simulink model "lqe_h"  (R2020b)
settings: Solver=VariableStepAuto  StartTime=0.0  StopTime=10.0  RelTol=1e-3
settings Model: Creator=leonk  LastModifiedBy=leonk

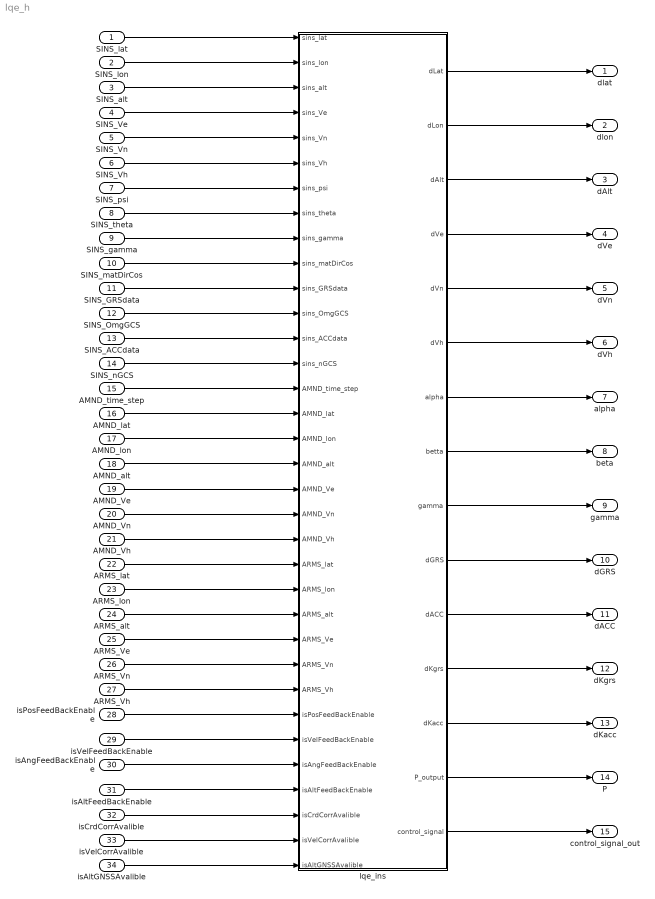
== system lqe_h ==
  SINS_lat : Inport  PortDimensions=1
  SINS_lon : Inport  Port=2  PortDimensions=1
  SINS_alt : Inport  Port=3  PortDimensions=1
  SINS_Ve : Inport  Port=4  PortDimensions=1
  SINS_Vn : Inport  Port=5  PortDimensions=1
  SINS_Vh : Inport  Port=6  PortDimensions=1
  SINS_psi : Inport  Port=7  PortDimensions=1
  SINS_theta : Inport  Port=8  PortDimensions=1
  SINS_gamma : Inport  Port=9  PortDimensions=1
  SINS_matDirCos : Inport  Port=10  PortDimensions=[3,3]
  SINS_GRSdata : Inport  Port=11  PortDimensions=[3,1]
  SINS_OmgGCS : Inport  Port=12  PortDimensions=[3,1]
  SINS_ACCdata : Inport  Port=13  PortDimensions=[3,1]
  SINS_nGCS : Inport  Port=14  PortDimensions=[3,1]
  AMND_time_step : Inport  Port=15  PortDimensions=1
  AMND_lat : Inport  Port=16  PortDimensions=1
  AMND_lon : Inport  Port=17  PortDimensions=1
  AMND_alt : Inport  Port=18  PortDimensions=1
  AMND_Ve : Inport  Port=19  PortDimensions=1
  AMND_Vn : Inport  Port=20  PortDimensions=1
  AMND_Vh : Inport  Port=21  PortDimensions=1
  ARMS_lat : Inport  Port=22  PortDimensions=1
  ARMS_lon : Inport  Port=23  PortDimensions=1
  ARMS_alt : Inport  Port=24  PortDimensions=1
  ARMS_Ve : Inport  Port=25  PortDimensions=1
  ARMS_Vn : Inport  Port=26  PortDimensions=1
  ARMS_Vh : Inport  Port=27  PortDimensions=1
  isPosFeedBackEnable : Inport  Port=28  PortDimensions=1
  isVelFeedBackEnable : Inport  Port=29  PortDimensions=1
  isAngFeedBackEnable : Inport  Port=30  PortDimensions=1
  isAltFeedBackEnable : Inport  Port=31  PortDimensions=1
  isCrdCorrAvalible : Inport  Port=32  PortDimensions=1
  isVelCorrAvalible : Inport  Port=33  PortDimensions=1
  isAltGNSSAvalible : Inport  Port=34  PortDimensions=1
  lqe_ins : MATLAB Function  TreatAsAtomicUnit=on
  dlat : Outport  PortDimensions=1  VectorParamsAs1DForOutWhenUnconnected=off
  dlon : Outport  Port=2  PortDimensions=1  VectorParamsAs1DForOutWhenUnconnected=off
  dAlt : Outport  Port=3  PortDimensions=1  VectorParamsAs1DForOutWhenUnconnected=off
  dVe : Outport  Port=4  PortDimensions=1  VectorParamsAs1DForOutWhenUnconnected=off
  dVn : Outport  Port=5  PortDimensions=1  VectorParamsAs1DForOutWhenUnconnected=off
  dVh : Outport  Port=6  PortDimensions=1  VectorParamsAs1DForOutWhenUnconnected=off
  alpha : Outport  Port=7  PortDimensions=1  VectorParamsAs1DForOutWhenUnconnected=off
  beta : Outport  Port=8  PortDimensions=1  VectorParamsAs1DForOutWhenUnconnected=off
  gamma : Outport  Port=9  PortDimensions=1  VectorParamsAs1DForOutWhenUnconnected=off
  dGRS : Outport  Port=10  PortDimensions=[3,1]  VectorParamsAs1DForOutWhenUnconnected=off
  dACC : Outport  Port=11  PortDimensions=[3,1]  VectorParamsAs1DForOutWhenUnconnected=off
  dKgrs : Outport  Port=12  PortDimensions=[3,1]  VectorParamsAs1DForOutWhenUnconnected=off
  dKacc : Outport  Port=13  PortDimensions=[3,1]  VectorParamsAs1DForOutWhenUnconnected=off
  P : Outport  Port=14  VectorParamsAs1DForOutWhenUnconnected=off
  control_signal_out : Outport  Port=15  PortDimensions=[4,1]  VectorParamsAs1DForOutWhenUnconnected=off
  wires:
  isAltFeedBackEnable/1 -> lqe_ins/31(isAltFeedBackEnable)
  lqe_ins/6(dVh) -> dVh/1
  AMND_lon/1 -> lqe_ins/17(AMND_lon)
  lqe_ins/9(gamma) -> gamma/1
  ARMS_Vn/1 -> lqe_ins/26(ARMS_Vn)
  lqe_ins/4(dVe) -> dVe/1
  SINS_alt/1 -> lqe_ins/3(sins_alt)
  isVelCorrAvalible/1 -> lqe_ins/33(isVelCorrAvalible)
  isCrdCorrAvalible/1 -> lqe_ins/32(isCrdCorrAvalible)
  lqe_ins/2(dLon) -> dlon/1
  AMND_Vn/1 -> lqe_ins/20(AMND_Vn)
  lqe_ins/5(dVn) -> dVn/1
  ARMS_Vh/1 -> lqe_ins/27(ARMS_Vh)
  lqe_ins/1(dLat) -> dlat/1
  AMND_alt/1 -> lqe_ins/18(AMND_alt)
  AMND_Vh/1 -> lqe_ins/21(AMND_Vh)
  lqe_ins/3(dAlt) -> dAlt/1
  ARMS_alt/1 -> lqe_ins/24(ARMS_alt)
  lqe_ins/8(betta) -> beta/1
  lqe_ins/13(dKacc) -> dKacc/1
  SINS_ACCdata/1 -> lqe_ins/13(sins_ACCdata)
  isPosFeedBackEnable/1 -> lqe_ins/28(isPosFeedBackEnable)
  lqe_ins/15(control_signal) -> control_signal_out/1
  AMND_time_step/1 -> lqe_ins/15(AMND_time_step)
  SINS_Ve/1 -> lqe_ins/4(sins_Ve)
  isVelFeedBackEnable/1 -> lqe_ins/29(isVelFeedBackEnable)
  AMND_Ve/1 -> lqe_ins/19(AMND_Ve)
  SINS_nGCS/1 -> lqe_ins/14(sins_nGCS)
  SINS_GRSdata/1 -> lqe_ins/11(sins_GRSdata)
  lqe_ins/10(dGRS) -> dGRS/1
  isAltGNSSAvalible/1 -> lqe_ins/34(isAltGNSSAvalible)
  SINS_Vh/1 -> lqe_ins/6(sins_Vh)
  ARMS_lon/1 -> lqe_ins/23(ARMS_lon)
  AMND_lat/1 -> lqe_ins/16(AMND_lat)
  isAngFeedBackEnable/1 -> lqe_ins/30(isAngFeedBackEnable)
  ARMS_Ve/1 -> lqe_ins/25(ARMS_Ve)
  ARMS_lat/1 -> lqe_ins/22(ARMS_lat)
  SINS_gamma/1 -> lqe_ins/9(sins_gamma)
  SINS_lat/1 -> lqe_ins/1(sins_lat)
  SINS_OmgGCS/1 -> lqe_ins/12(sins_OmgGCS)
  SINS_theta/1 -> lqe_ins/8(sins_theta)
  lqe_ins/12(dKgrs) -> dKgrs/1
  SINS_Vn/1 -> lqe_ins/5(sins_Vn)
  lqe_ins/11(dACC) -> dACC/1
  lqe_ins/14(P_output) -> P/1
  lqe_ins/7(alpha) -> alpha/1
  SINS_matDirCos/1 -> lqe_ins/10(sins_matDirCos)
  SINS_psi/1 -> lqe_ins/7(sins_psi)
  SINS_lon/1 -> lqe_ins/2(sins_lon)

== matlab function lqe_h/lqe_ins ==
  data: sins_lat input; sins_lon input; sins_alt input; sins_Ve input; sins_Vn input; sins_Vh input; sins_psi input; sins_theta input; sins_gamma input; sins_matDirCos input; sins_GRSdata input; sins_OmgGCS input; sins_ACCdata input; sins_nGCS input; AMND_time_step input; AMND_lat input; AMND_lon input; AMND_alt input; AMND_Ve input; AMND_Vn input; AMND_Vh input; ARMS_lat input; ARMS_lon input; ARMS_alt input; ARMS_Ve input; ARMS_Vn input; ARMS_Vh input; isPosFeedBackEnable input; isVelFeedBackEnable input; dLat output; dLon output; dAlt output; dVe output; dVn output; dVh output; alpha output; betta output; gamma output; dGRS output; dACC output; dKgrs output; dKacc output; isAngFeedBackEnable input; isAltFeedBackEnable input; P_output output; control_signal output; isCrdCorrAvalible input; isVelCorrAvalible input; isAltGNSSAvalible input
function [dLat,dLon,dAlt,dVe,dVn,dVh,alpha,betta,gamma,dGRS, dACC, dKgrs,dKacc,...
    P_output, control_signal]=...
    lqe_ins(...
    sins_lat, sins_lon, sins_alt, sins_Ve, sins_Vn, sins_Vh,sins_psi, sins_theta,...
    sins_gamma,sins_matDirCos, sins_GRSdata, sins_OmgGCS, sins_ACCdata,...
    sins_nGCS,...
    AMND_time_step,...
    AMND_lat, AMND_lon, AMND_alt, AMND_Ve, AMND_Vn, AMND_Vh,... 
    ARMS_lat, ARMS_lon,ARMS_alt, ARMS_Ve, ARMS_Vn, ARMS_Vh,...
    isPosFeedBackEnable, isVelFeedBackEnable, isAngFeedBackEnable, isAltFeedBackEnable,...
    isCrdCorrAvalible, isVelCorrAvalible, isAltGNSSAvalible)
   
    persistent LQE SINS AMND time 
    
    u = deg2rad(15/3600); 
    EARTH_A = 6378147;
    RO_1 = EARTH_A;
    RO_2 = EARTH_A;
    GRAVIT_CONST_EATRH = 3.9860e+14;
    EARTH_A = 6378147;
    SQR_OM_SH = (GRAVIT_CONST_EATRH/(EARTH_A*EARTH_A*EARTH_A));
    
    
    if isempty(LQE) 
        time = 0;
        LQE.Z = zeros(7,1);
        LQE.X = zeros(21,1);
        LQE.F = zeros(21,21);
        LQE.S = zeros(21,21);
        LQE.P = zeros(21,21);
        LQE.G = zeros(21,6);
        LQE.L = zeros(21,6);
        LQE.Q = zeros(6,6);
        LQE.K = zeros(21,7);
        LQE.R = zeros(7,7);
        LQE.H = zeros(7,21);
        LQE.prediction_step = 1/100;
        LQE.isPosFeedBackEnable = isPosFeedBackEnable;%0;%
        LQE.isVelFeedBackEnable = isVelFeedBackEnable;%0;%
        LQE.isAngFeedBackEnable = isAngFeedBackEnable;%0;%
        LQE.isAltFeedBackEnable = isAltFeedBackEnable;
        
        LQE.isCrdCorrAvalible   = 0;
        LQE.isVelCorrAvalible   = 0;
        LQE.isAltGNSSAvalible = 0;
        LQE.isCorrAvalible    = 0;
        
        LQE = init_PQ(LQE);
        
        SINS.lat   = 0;
        SINS.lon   = 0;
        SINS.alt   = 0;
        SINS.Ve    = 0;
        SINS.Vn    = 0;
        SINS.Vh    = 0;
        SINS.psi   = 0;
        SINS.theta = 0;
        SINS.gamma = 0;
        SINS.matDirCos = zeros(3,3);
        SINS.Omg_x = 0;
        SINS.Omg_y = 0;
        SINS.Omg_z = 0;
        SINS.Omg_e = 0;
        SINS.Omg_n = 0;
        SINS.Omg_h = 0;
        SINS.n_x   = 0;
        SINS.n_y   = 0;
        SINS.n_z   = 0;
        SINS.n_e   = 0;
        SINS.n_n   = 0;
        SINS.n_h   = 0;
        
        AMND.lat = 0;
        AMND.lon = 0;
        AMND.alt = 0;
        AMND.Ve  = 0;
        AMND.Vn  = 0;
        AMND.Vh = 0;
        AMND.lat_RMS = 0;
        AMND.lon_RMS = 0;
        AMND.alt_RMS = 0;
        AMND.Ve_RMS  = 0;
        AMND.Vn_RMS  = 0;
        AMND.Vh_RMS  = 0;
        
    end
    
    AMND.time_step = AMND_time_step;
%%%%%%%%%%%%%%%%%%%%%%%%%%%%%%%%%%%%%%%%%%%%%%%%%%%%%%%%%%%%%%%%%%%%%%%%%%%
%Определение размерности выходных данных
    dLat = 0; dLon = 0; dVe = 0; dVn = 0; alpha = 0; betta = 0; gamma = 0;
    dGRS=zeros(3,1); dACC=zeros(3,1); dKgrs=zeros(3,1); dKacc=zeros(3,1);
    
    P_output = zeros(length(LQE.P),1);
    
    control_signal = zeros(4,1);
%%%%%%%%%%%%%%%%%%%%%%%%%%%%%%%%%%%%%%%%%%%%%%%%%%%%%%%%%%%%%%%%%%%%%%%%%%%    
    LQE.isPosFeedBackEnable = isPosFeedBackEnable;
    LQE.isVelFeedBackEnable = isVelFeedBackEnable;
    LQE.isAngFeedBackEnable = isAngFeedBackEnable;
    LQE.isAltFeedBackEnable = isAltFeedBackEnable;
    
    LQE.isCrdCorrAvalible   = isCrdCorrAvalible;
    LQE.isVelCorrAvalible   = isVelCorrAvalible;
    LQE.isAltGNSSAvalible   = isAltGNSSAvalible;
    
    LQE.isCorrAvalible = 0;
    
    if isCrdCorrAvalible == 1 || isVelCorrAvalible == 1 || isAltGNSSAvalible== 1
        LQE.isCorrAvalible = 1;
    end
    
    
    SINS = parse_SINS(SINS, sins_lat, sins_lon, sins_alt, sins_Ve, sins_Vn,sins_Vh,...
        sins_psi, sins_theta, sins_gamma,...
        sins_matDirCos, sins_GRSdata, sins_OmgGCS, sins_ACCdata,sins_nGCS);
                    
    [AMND,LQE] = parse_AMND(AMND,LQE, AMND_lat, AMND_lon,AMND_alt,...
        AMND_Ve, AMND_Vn, AMND_Vh,...
        ARMS_lat, ARMS_lon, ARMS_alt,...
        ARMS_Ve, ARMS_Vn, ARMS_Vh,...
        isPosFeedBackEnable,isVelFeedBackEnable,isAngFeedBackEnable);
     
    LQE = update_GFL(LQE, SINS, RO_2, u, SQR_OM_SH);

% вычисление
        % Прогноз
        
 if time > 80
        
        LQE.X = LQE.F*LQE.X; 
        LQE.S = LQE.F*LQE.P*LQE.F' + LQE.L*LQE.Q*LQE.L';

        %Коррекция
        
        if  (LQE.isCorrAvalible == 1)
            LQE = update_H(LQE, SINS, AMND, RO_1, RO_2, EARTH_A); %Матрица H
            LQE = update_ZR(LQE,SINS,AMND,RO_1,RO_2);% вычисление новых Z и R

            LQE.K = (LQE.S*LQE.H')*inv(LQE.H*LQE.S*LQE.H' + LQE.R);
            LQE.P = (eye(size(LQE.P)) - LQE.K*LQE.H)*LQE.S;
            LQE.X = LQE.X + LQE.K*(LQE.Z - LQE.H*LQE.X);
        else
            LQE.P = LQE.S;
        end

        %if (LQE.P(5,5) < deg2rad(0.01)^2)||(LQE.P(6,6) < deg2rad(0.01)^2)
        %    LQE.P(5,5) = deg2rad(0.01)^2;
        %    LQE.P(6,6) = deg2rad(0.01)^2;
        %end
        %if (LQE.P(7,7) < deg2rad(0.05)^2)
        %    LQE.P(7,7) = deg2rad(0.05)^2;
        %end
       
    

else
    time = time + 0.01;
    LQE = init_PQ(LQE);
end
         
         
        [dLat,dLon,dAlt,dVe,dVn,dVh,alpha,betta,gamma,dGRS,dACC,dKgrs,dKacc,P_output,...
                      LQE, control_signal] = parse_back(LQE,SINS,AMND,EARTH_A);
end
%==========================================================================
function LQE = init_PQ(LQE)

    GRS_noise = deg2rad(0.15*1e-5)/60;
    ACC_noise = 1e-5;
    LQE.Q = diag([GRS_noise;GRS_noise;GRS_noise;... 
                    ACC_noise;ACC_noise;ACC_noise].^2)/LQE.prediction_step;

    LQE.P = diag([10;10;0.77;0.77;...                                      %lon,lat,Ve,Vn
                  deg2rad(0.1);deg2rad(0.1);deg2rad(0.5);%deg2rad(0.03);deg2rad(0.03);deg2rad(0.25);...            %alpha, betta, gamma
                  1.5*1e-6;1.5*1e-6;1.5*1e-6;...                           %dGRS
                  5*1e-4;5*1e-4;5*1e-4;...                                 %dKrgs
                  0.004;0.004;0.004;...                                    %dACC
                  3*1e-4;3*1e-4;3*1e-4;...                                 %dKacc
                  5;0.06].^2);                                             %alt, Vh
end
%==========================================================================
function [dLat,dLon,dAlt,dVe,dVn,dVh,alpha,betta,gamma,dGRS, dACC, dKgrs,dKacc,...
             P_output, LQE, control_signal] = parse_back(LQE,SINS,AMND,EARTH_A)
  
    dLon  = LQE.X(1,1)/(EARTH_A*cos(AMND.lat));                            %d_longitude
    dLat  = LQE.X(2,1)/(EARTH_A);                                          %d_latitude
    dAlt  = LQE.X(20,1);%%%%%%%%%%%%%%%%%%%%%%%%%%%%%%%%%%%%%%%%%%
    dVe   = LQE.X(3,1) - tan(AMND.lat)*dLon*LQE.X(1,1) - SINS.Omg_h*LQE.X(2,1);%d_Ve
    dVn   = LQE.X(4,1);                                                    %d_Vn
    dVh   = LQE.X(21,1);%%%%%%%%%%%%%%%%%%
    alpha = LQE.X(5,1) + (1/EARTH_A)*LQE.X(2);                             %d_alpha
    betta = LQE.X(6,1) - (1/EARTH_A)*LQE.X(1);                             %d_betta
    gamma = LQE.X(7,1) - (1/EARTH_A)*LQE.X(1)*tan(AMND.lat);               %d_gamma
    dGRS  = [LQE.X(8:10)];
    dKgrs = [LQE.X(11:13)];
    dACC  = [LQE.X(14:16)];
    dKacc = [LQE.X(17:19)];
    
    
    
    P_output = sqrt(diag(LQE.P));
    
    control_signal = zeros(4,1);

    if  (LQE.isPosFeedBackEnable == 1) && (LQE.isCorrAvalible == 1)
        LQE.X(1)  = 0;
        LQE.X(2)  = 0;
        control_signal(1) = 1;
    end
    if  (LQE.isVelFeedBackEnable == 1) && (LQE.isCorrAvalible == 1)
        LQE.X(3)  = 0;
        LQE.X(4)  = 0;
        control_signal(2) = 1;
    end
    if  (LQE.isAngFeedBackEnable == 1) && (LQE.isCorrAvalible == 1)
        LQE.X(5) = 0;
        LQE.X(6) = 0;
        LQE.X(7) = 0;
        control_signal(3) = 1;
    end
    if  (LQE.isAltFeedBackEnable == 1) && (LQE.isCorrAvalible == 1)
        LQE.X(20) = 0;       
        LQE.X(21) = 0;
        control_signal(4) = 1;
    end
    
end
%==========================================================================
function LQE = update_ZR(LQE,SINS,AMND,RO_1,RO_2)

    LQE.Z = zeros(size(LQE.Z));
    
    if (LQE.isCrdCorrAvalible == 1)
        LQE.Z(1)   = (SINS.lon - AMND.lon)*(RO_2*cos(AMND.lat));
        LQE.Z(2)   = (SINS.lat - AMND.lat)*RO_1;
    end
    if (LQE.isVelCorrAvalible == 1)
        LQE.Z(3)   = SINS.Ve - AMND.Ve;
        LQE.Z(4)   = SINS.Vn - AMND.Vn;
    end
    
    if LQE.isAltGNSSAvalible == 1
        LQE.Z(5)   = SINS.alt - AMND.alt;
        LQE.Z(6)   = SINS.Vh - AMND.Vh;
    end
    
        LQE.R(1,1) = (AMND.lon_RMS.^2)./AMND.time_step;
        LQE.R(2,2) = (AMND.lat_RMS.^2)./AMND.time_step;
        
        LQE.R(3,3) = (AMND.Ve_RMS.^2) ./AMND.time_step;
        LQE.R(4,4) = (AMND.Vn_RMS.^2) ./AMND.time_step;
        
        LQE.R(5,5) = (AMND.alt_RMS.^2)./AMND.time_step;
        LQE.R(6,6) = (AMND.Vh_RMS.^2) ./AMND.time_step;
        
        LQE.R(7,7) = 100;
end
%==========================================================================
function LQE = update_GFL(LQE, SINS, RO_2, u, omg_0)

    LQE.F = zeros(size(LQE.F));
    LQE.L = zeros(size(LQE.L));
    
    omg_e_dot = 0;
    omg_n_dot = 0;
    Omg_h_dot =1/RO_2*(u*cos(SINS.lat)*SINS.Ve + SINS.n_e*tan(SINS.lat)+...
           + SINS.Vh*SINS.Omg_h + SINS.Ve*SINS.Vn/(RO_2*cos(SINS.lat).^2));
       
    LQE.G(3,4) = SINS.matDirCos(1,1);
    LQE.G(3,5) = SINS.matDirCos(1,2);
    LQE.G(3,6) = SINS.matDirCos(1,3);
    
    LQE.G(4,4) = SINS.matDirCos(2,1);
    LQE.G(4,5) = SINS.matDirCos(2,2);
    LQE.G(4,6) = SINS.matDirCos(2,3);
    
    LQE.G(21,4) = SINS.matDirCos(3,1);%%%%%%%%%%%%%%%%%%%%%%%%%%%%%%
    LQE.G(21,5) = SINS.matDirCos(3,2);%%%%%%%%%%%%%%%%%%%%%%%%%%%%%%
    LQE.G(21,6) = SINS.matDirCos(3,3);%%%%%%%%%%%%%%%%%%%%%%%%%%%%%%
    
    LQE.G(5,1) = SINS.matDirCos(1,1);
    LQE.G(5,2) = SINS.matDirCos(1,2);
    LQE.G(5,3) = SINS.matDirCos(1,3);
    
    LQE.G(6,1) = SINS.matDirCos(2,1);
    LQE.G(6,2) = SINS.matDirCos(2,2);
    LQE.G(6,3) = SINS.matDirCos(2,3);

    LQE.G(7,1) = SINS.matDirCos(3,1);
    LQE.G(7,2) = SINS.matDirCos(3,2);
    LQE.G(7,3) = SINS.matDirCos(3,3);
         
    LQE.F(1,3) = 1; 
    LQE.F(2,4) = 1;
    
    LQE.F(3,1) = -omg_0.^2 + SINS.Omg_n.^2+SINS.Omg_h.^2;
    LQE.F(3,2) = Omg_h_dot-SINS.Omg_e*SINS.Omg_n;
    
    LQE.F(3,4) =  2*SINS.Omg_h;
    
    LQE.F(3,20) = -(omg_n_dot + SINS.Omg_e*SINS.Omg_h);%%%%%%%%%%%%%%%%%%%%%%
    LQE.F(3,21) = -2*SINS.Omg_n;                       %%%%%%%%%%%%%%%%%%%%%% 
    %Дмитроченко  %Антонов+
    LQE.F(3,6) = -SINS.n_h;%%%%%%%%%%%%%%%%%%%%%% 
    LQE.F(3,7) =  SINS.n_n;%%%%%%%%%%%%%%%%%%%%%% 

    LQE.F(4,2) = -omg_0.^2 + SINS.Omg_e.^2+SINS.Omg_h.^2;
    LQE.F(4,3) = -LQE.F(3,4);
    
    LQE.F(4,5) =  SINS.n_h;%SINS.n_h%%%%%%%%%%%%%%%%%%%%% 
    LQE.F(4,7) = -SINS.n_e;%SINS.n_e%%%%%%%%%%%%%%%%%%%%% 
    
    LQE.F(4,20) = omg_e_dot - SINS.Omg_n*SINS.Omg_h;%%%%%%%%%%%%%%%%%%%%%%%%%%%%%
    LQE.F(4,21) = 2*SINS.Omg_e;
    
    LQE.F(3,14) = SINS.matDirCos(1,1);
    LQE.F(3,15) = SINS.matDirCos(1,2);
    LQE.F(3,16) = SINS.matDirCos(1,3);
    
    LQE.F(3,17) = SINS.n_x*SINS.matDirCos(1,1);
    LQE.F(3,18) = SINS.n_y*SINS.matDirCos(1,2);
    LQE.F(3,19) = SINS.n_z*SINS.matDirCos(1,3);
    
    LQE.F(4,14) = SINS.matDirCos(2,1);
    LQE.F(4,15) = SINS.matDirCos(2,2);
    LQE.F(4,16) = SINS.matDirCos(2,3);
    
    LQE.F(4,17) = SINS.n_x*SINS.matDirCos(2,1);
    LQE.F(4,18) = SINS.n_y*SINS.matDirCos(2,2);
    LQE.F(4,19) = SINS.n_z*SINS.matDirCos(2,3);

    LQE.F(5,5)  = 0;
    LQE.F(5,6)  = SINS.Omg_h;%z
    LQE.F(5,7)  =-SINS.Omg_n;%y
    
    LQE.F(6,5)  =-SINS.Omg_h;%z
    LQE.F(6,6)  = 0;
    LQE.F(6,7)  = SINS.Omg_e;%x
    
    LQE.F(7,5)  = SINS.Omg_n;%y
    LQE.F(7,6)  =-SINS.Omg_e;%x
    LQE.F(7,7) = 0;
    
    LQE.F(5,8)   = SINS.matDirCos(1,1);
    LQE.F(5,9)   = SINS.matDirCos(1,2);
    LQE.F(5,10)  = SINS.matDirCos(1,3);
    
    LQE.F(6,8)   = SINS.matDirCos(2,1);
    LQE.F(6,9)   = SINS.matDirCos(2,2);
    LQE.F(6,10)  = SINS.matDirCos(2,3);
    
    LQE.F(7,8)  = SINS.matDirCos(3,1);
    LQE.F(7,9)  = SINS.matDirCos(3,2);
    LQE.F(7,10) = SINS.matDirCos(3,3);
    
    
    LQE.F(20,21) = 1;
    
    LQE.F(21,1)  =  omg_n_dot -SINS.Omg_e*SINS.Omg_h; 
    LQE.F(21,3)  =  2*SINS.Omg_n;
    LQE.F(21,2)  = -(omg_e_dot + SINS.Omg_n*SINS.Omg_h);
    LQE.F(21,4)  =  2*SINS.Omg_e;
    LQE.F(21,5)  = -SINS.n_n;%%%%%%%%%%%%%%%%%%
    LQE.F(21,6)  =  SINS.n_e;%%%%%%%%%%%%%%%%%%%

    LQE.F(21,14) = SINS.matDirCos(3,1);
    LQE.F(21,15) = SINS.matDirCos(3,2);
    LQE.F(21,16) = SINS.matDirCos(3,3);
    
    LQE.F(21,17) = SINS.n_x*SINS.matDirCos(3,1);
    LQE.F(21,18) = SINS.n_y*SINS.matDirCos(3,2);
    LQE.F(21,19) = SINS.n_z*SINS.matDirCos(3,3);
    
    LQE.F(21,20) =  2*omg_0.^2 + SINS.Omg_e.^2 + SINS.Omg_n.^2;%&&&&&&&&&&&&&&&&&&&&&&&
       
    
    
    
    LQE.F = eye(size(LQE.F)) + LQE.F.*LQE.prediction_step;
    LQE.L = LQE.F*LQE.G.*LQE.prediction_step;
end
%==========================================================================
function SINS = parse_SINS(SINS, sins_lat, sins_lon, sins_alt, sins_Ve, sins_Vn,sins_Vh,...
         sins_psi, sins_theta, sins_gamma,...
         sins_matDirCos, sins_GRSdata, sins_OmgGCS, sins_ACCdata,sins_nGCS)

	SINS.lat   = sins_lat;
    SINS.lon   = sins_lon;
    SINS.alt   = sins_alt;
    SINS.Ve    = sins_Ve;
    SINS.Vn    = sins_Vn;
    SINS.Vh    = sins_Vh;
    SINS.psi   = sins_psi;
    SINS.theta = sins_theta;
    SINS.gamma = sins_gamma;
    SINS.matDirCos = sins_matDirCos;
    
    SINS.Omg_x = sins_GRSdata(1);
    SINS.Omg_y = sins_GRSdata(2);
    SINS.Omg_z = sins_GRSdata(3);
    
    SINS.Omg_e = sins_OmgGCS(1);
    SINS.Omg_n = sins_OmgGCS(2);
    SINS.Omg_h = sins_OmgGCS(3);
    
    SINS.n_x = sins_ACCdata(1);
    SINS.n_y = sins_ACCdata(2);
    SINS.n_z = sins_ACCdata(3);
    
    SINS.n_e = sins_nGCS(1);
    SINS.n_n = sins_nGCS(2);
    SINS.n_h = sins_nGCS(3);
    
end
%==========================================================================
function [AMND,LQE] = parse_AMND(AMND,LQE, AMND_lat, AMND_lon,AMND_alt,...
            AMND_Ve, AMND_Vn, AMND_Vh, ARMS_lat, ARMS_lon, ARMS_alt,...
            ARMS_Ve, ARMS_Vn, ARMS_Vh,...
            isPosFeedBackEnable,isVelFeedBackEnable,isAngFeedBackEnable)

    AMND.lat = AMND_lat;
    AMND.lon = AMND_lon;
    AMND.alt = AMND_alt;
    AMND.Ve  = AMND_Ve;
    AMND.Vn  = AMND_Vn;
    AMND.Vh  = AMND_Vh;
        
    AMND.lat_RMS = ARMS_lat;
    AMND.lon_RMS = ARMS_lon;
    AMND.alt_RMS = ARMS_alt;
    AMND.Ve_RMS  = ARMS_Ve;
    AMND.Vn_RMS  = ARMS_Vn;
    AMND.Vh_RMS  = ARMS_Vh; 
    
    LQE.isPosFeedBackEnable = isPosFeedBackEnable;
    LQE.isVelFeedBackEnable = isVelFeedBackEnable;
    LQE.isAngFeedBackEnable = isAngFeedBackEnable;
    
end
%==========================================================================
function LQE = update_H(LQE, SINS, AMND, RO_1, RO_2, EARTH_A)

    LQE.H = zeros(size(LQE.H)); 
    
    if LQE.isCrdCorrAvalible == 1
        LQE.H(1,1) = 1;                                                    % calculate dLat&dLon as meters
        LQE.H(2,2) = 1;                                                    
    end
    
    if LQE.isVelCorrAvalible == 1
        LQE.H(3,1) = -(SINS.Vh/RO_2 + SINS.Omg_e*tan(AMND.lat));
        LQE.H(3,2) = -SINS.Omg_h;
        LQE.H(3,3) =  1;
        LQE.H(4,1) = -SINS.Vh/RO_1;
        LQE.H(4,4) = 1;
    end
    
    if LQE.isAltGNSSAvalible == 1
        LQE.H(5,20) = 1;%%%%%%%%%%%%%%%%%%%%%                                                    
        LQE.H(6,21) = 1;                     %%%%%%%%%%%%%%%%%%%%%%%%%%%                               
    end
   % if LQE.isAltRVAvalible == 1
   %     LQE.H(20,20) = 1;                                                    % calculate dLat&dLon as meters
   %     LQE.H(21,21) = 1;                                                    
   % end
    
end
